simulink library "Interface"  (R2018b)
settings: Solver=VariableStepAuto  StartTime=0.0  StopTime=10.0  RelTol=1e-3
settings Model: ModifiedHistory=% Copyright 2018 The MathWorks, Inc.  Creator=sdupertu  LastModifiedBy=sdupertu
settings DebuggingCC: LibraryContextMissingDiagnostic=none
settings SFSimCC: SimCustomHeaderCode="#include \"ParkingMeterMemory.h\""  SimUserSources=ParkingMeterMemory.c  SimUserIncludeDirs=..\Interface_C_files
settings RTWCC: RTWUseLocalCustomCode=off

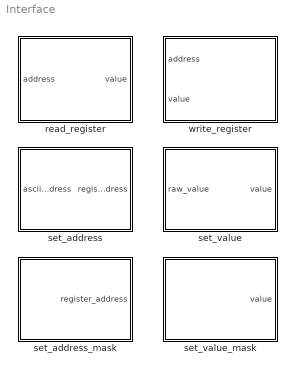
== system Interface ==
  read_register : Subsystem  Variant=on  VariantControl=Variant1
  set_address : Subsystem
  set_address_mask : Subsystem  mask{RegisterAddress=[0 0 0 0 0 0]}
      mask prompts: RegisterAddress "Address Array in ASCII code"
  set_value : Subsystem
  set_value_mask : Subsystem  mask{raw_value=0}
      mask prompts: raw_value "Value in uint8"
  write_register : Subsystem  Variant=on  VariantControl=Variant1

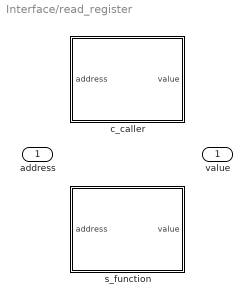
== system Interface/read_register ==
  "address " : Inport
  c_caller : Subsystem  VariantControl=SRC
  s_function : Subsystem  VariantControl=MEX
  " value" : Outport

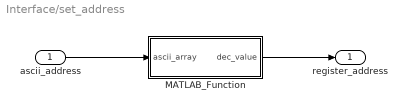
== system Interface/set_address ==
  ascii_address : Inport  OutDataTypeStr=uint8
  MATLAB_Function : MATLAB Function  TreatAsAtomicUnit=on
  register_address : Outport
  wires:
  MATLAB_Function/1(dec_value) -> register_address/1
  ascii_address/1 -> MATLAB_Function/1(ascii_array)

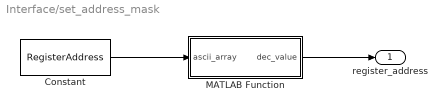
== system Interface/set_address_mask ==
  Constant : Constant  Value=RegisterAddress  VectorParams1D=off  OutDataTypeStr=uint8
  MATLAB Function : MATLAB Function  TreatAsAtomicUnit=on
  register_address : Outport
  wires:
  MATLAB Function/1(dec_value) -> register_address/1
  Constant/1 -> MATLAB Function/1(ascii_array)

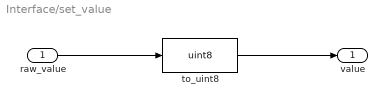
== system Interface/set_value ==
  raw_value : Inport
  to_uint8 : DataTypeConversion  OutMin=0  OutMax=255  OutDataTypeStr=uint8
  value : Outport
  wires:
  raw_value/1 -> to_uint8/1
  to_uint8/1 -> value/1

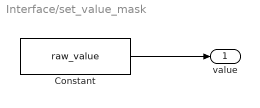
== system Interface/set_value_mask ==
  Constant : Constant  Value=raw_value  OutMin=0  OutMax=255  OutDataTypeStr=uint8
  value : Outport
  wires:
  Constant/1 -> value/1

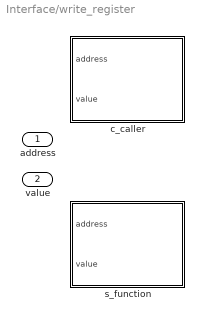
== system Interface/write_register ==
  "address " : Inport
  "value " : Inport  Port=2
  c_caller : Subsystem  VariantControl=SRC
  s_function : Subsystem  VariantControl=MEX

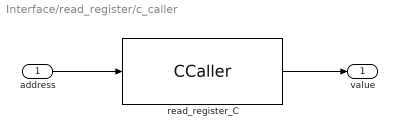
== system Interface/read_register/c_caller ==
  address : Inport
  read_register_C : CCaller  FunctionName=read_register  PortSpecificationStruct="%)30     .    4 ,   8    (     @         %    \"     (    !     0         %  0 \"0    $    V    07)G3F%M90  4&]R=$YA;64 4V-O<&4     26YD97@     5'EP90      4VEZ90         .    ,     8    (    !          %    \"     $    #     0         0  , ;W5T  X    P    !@    @    $          4    (     0    ,    !         !   P!O=70 #@   #@    &    \"     0         !0    @    !    !@    $         $     8   !/=71P=70   X    X    !@    @    &          4    (     0    $    !          D    (               .    .     8    (    !          %    \"     $    %     0         0    !0   '5I;G0X    #@   #     &    \"     0         !0    @    !     0    $         $  ! #$    .    .     8    (    !          %    \"     $    '     0         0    !P   &%D9')E<W, #@   #@    &    \"     0         !0    @    !    !P    $         $     <   !A9&1R97-S  X    X    !@    @    $          4    (     0    4    !         !     %    26YP=70    .    .     8    (    !@         %    \"     $    !     0         )    \"               #@   #@    &    \"     0         !0    @    !    !@    $         $     8   !U:6YT,38   X    P    !@    @    $          4    (     0    $    !         !   0 Q"
  value : Outport
  wires:
  read_register_C/1 -> value/1
  address/1 -> read_register_C/1

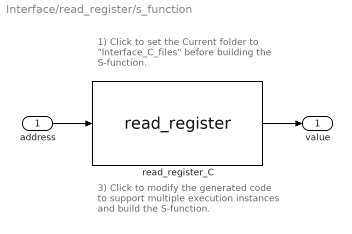
== system Interface/read_register/s_function ==
  note: 1) Click to set the Current folder to "Interface_C_files" before building the S-function.
  note: 3) Click to modify the generated code to support multiple execution instances and build the S-function.
  address : Inport
  read_register_C : S-Function  InitFcn=try, set_param(gcb,'FunctionName','read_register'), end  FunctionName=read_register  SFunctionModules=read_register_wrapper  SFunctionDeploymentMode=off  EnableBusSupport=off  mask(S-Function Builder){}
      mask help: Simulink:masks:SFunctionBuilder_MD
      mask init:
      | val = [[.9  0.75 0.75 1 1 .9 .9 1]',[1 1 0.75 0.75 .9 .9 1 .9]'];try , sys = get_param(gcb,'SfunBuilderFcnName');if isempty(sys), sys = get_param(gcb,'FunctionName'); end,catch, sys = get_param(gcb,'FunctionName'); end
      settings: CopyFcn=set_param(gcbh,'LinkStatus','none')  PreSaveFcn=try, set_param(gcb,'FunctionName','read_register'), end  OpenFcn=sfunctionwizard(gcbh)
      mask Display:
      | text(0.02,0.82,'2) Double click on the S-Function\nblock and click "Save" to generate\nthe needed files.');
      | plot(val(:,1),val(:,2)),disp(sys), port_label('input',1,'address'), port_label('output',1,'value')
  value : Outport
  wires:
  address/1 -> read_register_C/1
  read_register_C/1 -> value/1

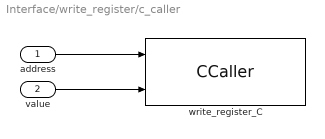
== system Interface/write_register/c_caller ==
  "address " : Inport
  "value " : Inport  Port=2
  write_register_C : CCaller  FunctionName=write_register  PortSpecificationStruct="%)30     .    8 ,   8    (     @         %    \"     (    !     0         %  0 \"0    $    V    07)G3F%M90  4&]R=$YA;64 4V-O<&4     26YD97@     5'EP90      4VEZ90         .    .     8    (    !          %    \"     $    '     0         0    !P   &%D9')E<W, #@   #@    &    \"     0         !0    @    !    !P    $         $     <   !A9&1R97-S  X    X    !@    @    $          4    (     0    4    !         !     %    26YP=70    .    .     8    (    !@         %    \"     $    !     0         )    \"               #@   #@    &    \"     0         !0    @    !    !@    $         $     8   !U:6YT,38   X    P    !@    @    $          4    (     0    $    !         !   0 Q    #@   #@    &    \"     0         !0    @    !    !0    $         $     4   !V86QU90    X    X    !@    @    $          4    (     0    4    !         !     %    =F%L=64    .    .     8    (    !          %    \"     $    %     0         0    !0   $EN<'5T    #@   #@    &    \"     8         !0    @    !     0    $         \"0    @           #P/PX    X    !@    @    $          4    (     0    4    !         !     %    =6EN=#@    .    ,     8    (    !          %    \"     $    !     0         0  $ ,0"
  wires:
  "value "/1 -> write_register_C/2
  "address "/1 -> write_register_C/1

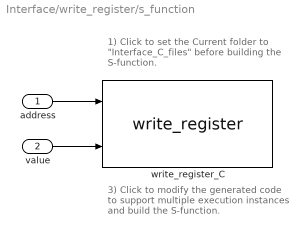
== system Interface/write_register/s_function ==
  note: 1) Click to set the Current folder to "Interface_C_files" before building the S-function.
  note: 3) Click to modify the generated code to support multiple execution instances and build the S-function.
  address : Inport
  value : Inport  Port=2
  write_register_C : S-Function  InitFcn=try, set_param(gcb,'FunctionName','write_register'), end  FunctionName=write_register  SFunctionModules=write_register_wrapper  SFunctionDeploymentMode=off  EnableBusSupport=off  mask(S-Function Builder){}
      mask help: Simulink:masks:SFunctionBuilder_MD
      mask init: same as Interface/read_register/s_function/read_register_C
      settings: CopyFcn=set_param(gcbh,'LinkStatus','none')  PreSaveFcn=try, set_param(gcb,'FunctionName','write_register'), end  OpenFcn=sfunctionwizard(gcbh)
      mask Display:
      | text(0.02,0.82,'2) Double click on the S-Function\nblock and click "Save" to generate\nthe needed files.');
      | plot(val(:,1),val(:,2)),disp(sys), port_label('input',1,'address'), port_label('input',2,'value')
  wires:
  address/1 -> write_register_C/1
  value/1 -> write_register_C/2

== matlab function Interface/set_address_mask/MATLAB Function ==
  data: ascii_array input; dec_value output
function dec_value  = char2dec(ascii_array)
%%%%%%%%%%%%%%%%%%%%%%%%%%%%%%%%%%%%%%%%%%%%%%%%%%%%%%%%%%%%%%%%%%%%%%%%%%%%%%%%
% Function char2dec()
% Goal  : Convert a number encoded in binary or hexadecimal base to decimal
% IN    : - char_sequence: char representation of the encoded value with the
%           prefix for the encoding format: '0b' = binary and '0x' = hexadecimal
% IN/OUT: -
% OUT   : - dec_value: decimal representation of the char sequence
%%%%%%%%%%%%%%%%%%%%%%%%%%%%%%%%%%%%%%%%%%%%%%%%%%%%%%%%%%%%%%%%%%%%%%%%%%%%%%%%
%#codegen
  % Local constants declaration
  FORMAT_LENGTH = 2; % Number of chars for the format of the encoded value
  HEXA_PER_BYTE = 2; % Number of hexa digit per byte
  % Convert ASCII input into char for further processing
  char_sequence = char(ascii_array);
  % Get the input number format of the value to store
  char_format = char_sequence(1:FORMAT_LENGTH);
  % Get the encoded value to store
  char_value = char_sequence(FORMAT_LENGTH+1:end);
  % Get the length of the encode value
  length_value = length(char_value);

  % Apply the right conversion based on the data format
  switch (char_format)
    case '0b'
      % Convert the binary char input to a UINT8 with LSB first
      dec_value = uint16(bi2de(char_value == '1', 'left-msb'));
    case '0x'
      if (length_value == HEXA_PER_BYTE)
        % Convert the hexa char input to a UINT8
        dec_value = uint16(hex2dec(char_value));
      elseif (length_value == 2*HEXA_PER_BYTE)
        % Convert the hexa char input to a UINT16
        dec_value = uint16(hex2dec(char_value));
      else
        dec_value = uint16(0);
        fprintf('Unsupported hexadecimal size.\n');
      end
    otherwise
      dec_value = uint16(0);
      fprintf('Unknown format number.\n');
  end
end

== matlab function Interface/set_address/MATLAB_Function ==
  data: ascii_array input; dec_value output
function dec_value  = char2dec(ascii_array)
%%%%%%%%%%%%%%%%%%%%%%%%%%%%%%%%%%%%%%%%%%%%%%%%%%%%%%%%%%%%%%%%%%%%%%%%%%%%%%%%
% Function char2dec()
% Goal  : Convert a number encoded in binary or hexadecimal base to decimal
% IN    : - char_sequence: char representation of the encoded value with the
%           prefix for the encoding format: '0b' = binary and '0x' = hexadecimal
% IN/OUT: -
% OUT   : - dec_value: decimal representation of the char sequence
%%%%%%%%%%%%%%%%%%%%%%%%%%%%%%%%%%%%%%%%%%%%%%%%%%%%%%%%%%%%%%%%%%%%%%%%%%%%%%%%
%#codegen
  % Local constants declaration
  FORMAT_LENGTH = 2; % Number of chars for the format of the encoded value
  HEXA_PER_BYTE = 2; % Number of hexa digit per byte
  % Convert ASCII input into char for further processing
  char_sequence = char(ascii_array);
  % Get the input number format of the value to store
  char_format = char_sequence(1:FORMAT_LENGTH);
  % Get the encoded value to store
  char_value = char_sequence(FORMAT_LENGTH+1:end);
  % Get the length of the encode value
  length_value = length(char_value);

  % Apply the right conversion based on the data format
  switch (char_format)
    case '0b'
      % Convert the binary char input to a UINT8 with LSB first
      dec_value = uint16(bi2de(char_value == '1',2,'left-msb'));
    case '0x'
      if (length_value == HEXA_PER_BYTE)
        % Convert the hexa char input to a UINT8
        dec_value = uint16(hex2dec(char_value));
      elseif (length_value == 2*HEXA_PER_BYTE)
        % Convert the hexa char input to a UINT16
        dec_value = uint16(hex2dec(char_value));
      else
        dec_value = uint16(0);
        fprintf('Unsupported hexadecimal size.\n');
      end
    otherwise
      dec_value = uint16(0);
      fprintf('Unknown format number.\n');
  end
end
